simulink model "QuarterCar"  (R2021b)
settings: Solver=ode1  StartTime=0.0  StopTime=inf  FixedStep=0.001  RelTol=1e-3
model workspace (MAT data in the model file):
  Sig = Simulink.Signal
  Sig.DataType = 'auto'
  Sig.Dimensions = -1
  Sig.DimensionsMode = 'auto'
  Sig.Complexity = 'auto'
  Sig.SampleTime = -1
  Sig.SamplingMode = 'auto'
  Sig1 = Simulink.Signal
  Sig1.DataType = 'auto'
  Sig1.Dimensions = -1
  Sig1.DimensionsMode = 'auto'
  Sig1.Complexity = 'auto'
  Sig1.SampleTime = -1
  Sig1.SamplingMode = 'auto'
  Sig2 = Simulink.Signal
  Sig2.DataType = 'auto'
  Sig2.Dimensions = -1
  Sig2.DimensionsMode = 'auto'
  Sig2.Complexity = 'auto'
  Sig2.SampleTime = -1
  Sig2.SamplingMode = 'auto'
undefined symbols (not defined in the file): c_susp, c_tire, g, k_susp, k_tire, m_sprung, m_unsprung, X_sprung0, X_unsprung0
settings Model: Creator=jalfonso  LastModifiedBy=au602135
settings SolverCC: AlgebraicLoopSolver=TrustRegion
settings DataIOCC: ReturnWorkspaceOutputs=off
settings DebuggingCC: SFMachineParentedDataDiag=warning  ArithmeticOperatorsInVariantConditions=warning
settings SFSimCC: SimUseLocalCustomCode=off  CustomCodeUndefinedFunction=UseInterfaceOnly
settings RTWCC: RTWUseLocalCustomCode=off
settings CodeAppCC: StateflowObjectComments=on

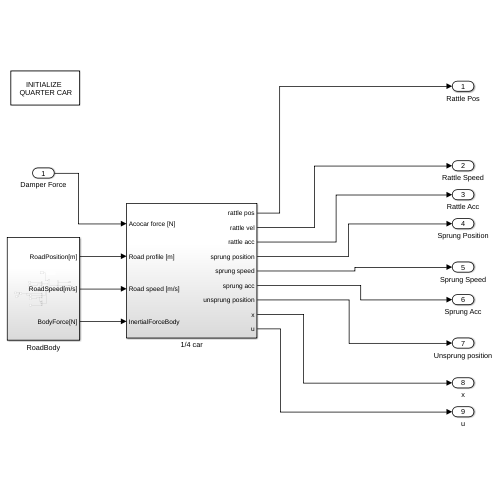
[thumbnail: Simulink's stored preview of the top-level diagram]
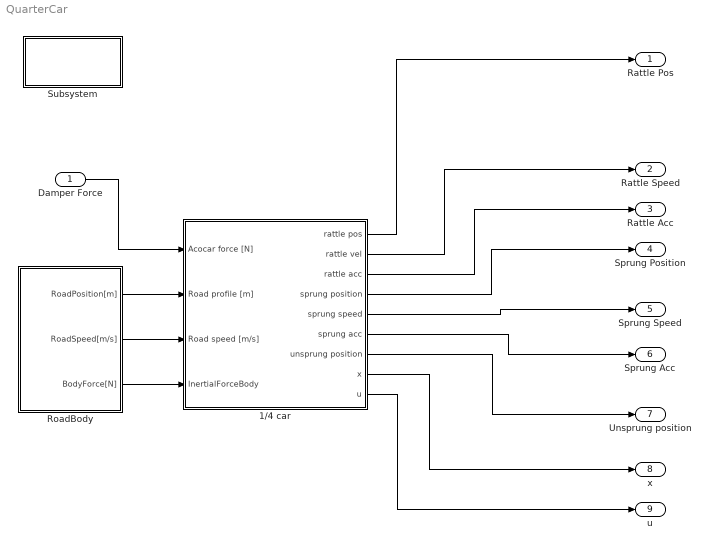
== system QuarterCar ==
  Damper Force : Inport
  1/4 car : Subsystem
  RoadBody : Subsystem
  Subsystem : Subsystem
      settings: OpenFcn=|
      | k_tire = 225400;  %200000 in literature
      | c_tire = 100;        % Estimated. In literatures 6N
      | k_susp =  25000;  % 15000 in literature
      | c_susp = 400;       %1429 Ns/m in literature
      | g = 0 % 9.8; Removed to avoid initialization problems
      | m_unsprung = 66;
      | m_sprung = 449.25;
      | X_sprung0  = .5;
      | X_unsprung0  = .1;
      | delayTimeCarToDamper =  0.002;
      | %InitQuarterCarCompensatorScript;
      | %Amplitude =.01;
      mask Display: disp('INITIALIZE \n QUARTER CAR')
  Rattle Pos : Outport
  Rattle Speed : Outport  Port=2
  Rattle Acc : Outport  Port=3
  Sprung Position : Outport  Port=4
  Sprung Speed : Outport  Port=5
  Sprung Acc : Outport  Port=6
  Unsprung position : Outport  Port=7
  x : Outport  Port=8
  u : Outport  Port=9
  wires:
  RoadBody/1(RoadPosition[m]) -> 1/4 car/2(Road profile [m])
  RoadBody/3(BodyForce[N]) -> 1/4 car/4(InertialForceBody)
  RoadBody/2(RoadSpeed[m/s]) -> 1/4 car/3(Road speed [m/s])
  Damper Force/1 -> 1/4 car/1(Acocar force [N])
  1/4 car/1(rattle pos) -> Rattle Pos/1
  1/4 car/2(rattle vel) -> Rattle Speed/1
  1/4 car/3(rattle acc) -> Rattle Acc/1
  1/4 car/4(sprung position) -> Sprung Position/1
  1/4 car/5(sprung speed) -> Sprung Speed/1
  1/4 car/6(sprung acc) -> Sprung Acc/1
  1/4 car/7(unsprung position) -> Unsprung position/1
  1/4 car/8(x) -> x/1
  1/4 car/9(u) -> u/1

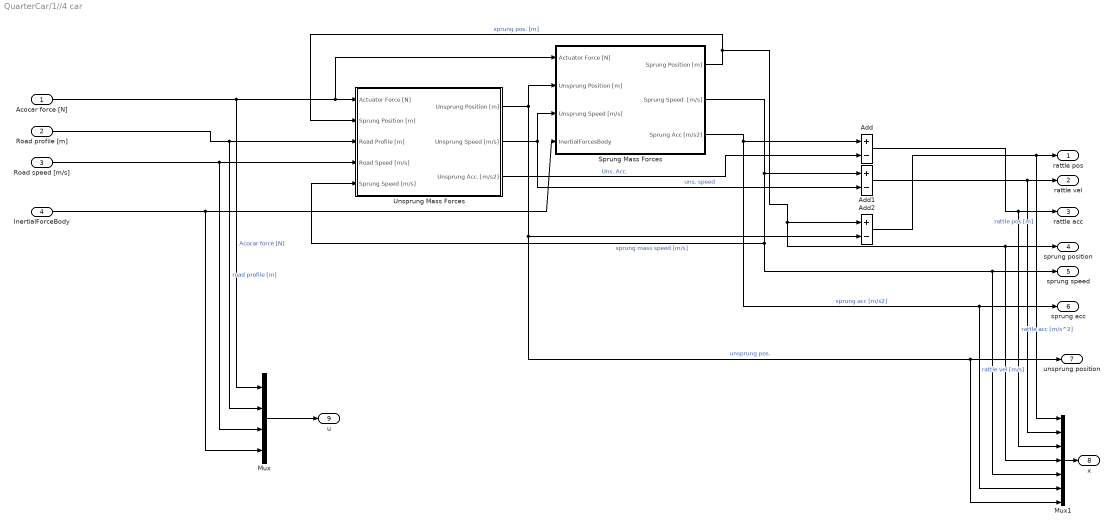
== system QuarterCar/1//4 car ==
  Acocar force [N] : Inport
  Road profile [m] : Inport  Port=2
  Road speed [m/s] : Inport  Port=3
  InertialForceBody : Inport  Port=4
  Add : Sum  Inputs=+-
  Add1 : Sum  Inputs=+-
  Add2 : Sum  Inputs=+-
  Mux : Mux
  Mux1 : Mux  Inputs=7
  Sprung Mass Forces : Subsystem
  Unsprung Mass Forces : Subsystem
  rattle pos : Outport
  rattle vel : Outport  Port=2
  rattle acc : Outport  Port=3
  sprung position : Outport  Port=4
  sprung speed : Outport  Port=5
  sprung acc : Outport  Port=6
  unsprung position : Outport  Port=7
  x : Outport  Port=8
  u : Outport  Port=9
  wires:
  Acocar force [N]/1 -> Mux/1, Sprung Mass Forces/1(Actuator Force [N]), Unsprung Mass Forces/1(Actuator Force [N])  "Acocar force [N]"
  Unsprung Mass Forces/1(Unsprung Position [m]) -> Sprung Mass Forces/2(Unsprung Position [m]), Mux1/7, unsprung position/1, Add2/2  "unsprung pos."
  Unsprung Mass Forces/2(Unsprung Speed [m/s]) -> Sprung Mass Forces/3(Unsprung Speed [m/s]), Add1/2  "uns. speed"
  Sprung Mass Forces/2(Sprung Speed  [m/s]) -> Mux1/5, sprung speed/1, Unsprung Mass Forces/5(Sprung Speed [m/s]), Add1/1  "sprung mass speed [m/s]"
  Sprung Mass Forces/1(Sprung Position [m]) -> Add2/1, Mux1/4, sprung position/1, Unsprung Mass Forces/2(Sprung Position [m])  "sprung pos. [m]"
  Road profile [m]/1 -> Mux/2, Unsprung Mass Forces/3(Road Profile [m])  "road profile [m]"
  Sprung Mass Forces/3(Sprung Acc [m/s2]) -> Mux1/6, sprung acc/1, Add/1  "sprung acc [m/s2]"
  Unsprung Mass Forces/3(Unsprung Acc. [m/s2]) -> Add/2  "Uns. Acc."
  Add/1 -> Mux1/3, rattle acc/1  "rattle acc [m/s^2]"
  Add2/1 -> Mux1/1, rattle pos/1  "rattle pos [m]"
  Add1/1 -> Mux1/2, rattle vel/1  "rattle vel [m/s]"
  Road speed [m/s]/1 -> Mux/3, Unsprung Mass Forces/4(Road Speed [m/s])
  InertialForceBody/1 -> Mux/4, Sprung Mass Forces/4(InertialForcesBody)
  Mux/1 -> u/1
  Mux1/1 -> x/1

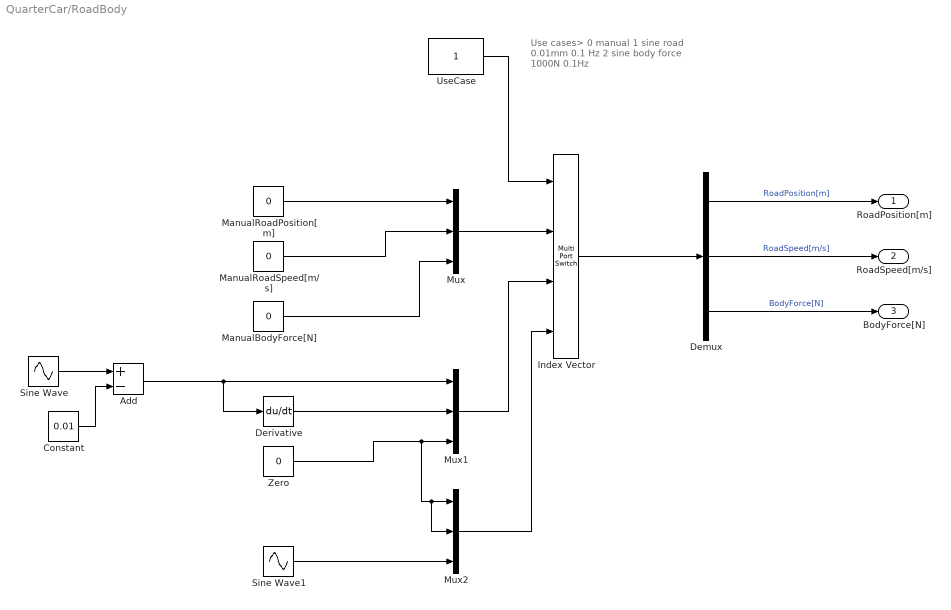
== system QuarterCar/RoadBody ==
  note: Use cases>
      |  0  manual
      | 1 sine road 0.01mm 0.1 Hz
      | 2 sine body force 1000N 0.1Hz
  Add : Sum  Inputs=+-
  Constant : Constant  Value=0.01
  Demux : Demux  Outputs=3
  Derivative : Derivative
  Index Vector : MultiPortSwitch  DataPortOrder=Zero-based contiguous  zeroidx=on
  ManualBodyForce[N] : Constant  Value=0
  ManualRoadPosition[m] : Constant  Value=0
  ManualRoadSpeed[m/s] : Constant  Value=0
  Mux : Mux  Inputs=3
  Mux1 : Mux  Inputs=3
  Mux2 : Mux  Inputs=3
  Sine Wave : Sin  Amplitude=0.01  Frequency=5*(2*pi)  Phase=pi/2  SampleTime=0
  Sine Wave1 : Sin  Amplitude=0.01  Frequency=0.2*pi  SampleTime=0
  UseCase : Constant
  Zero : Constant  Value=0
  RoadPosition[m] : Outport
  RoadSpeed[m/s] : Outport  Port=2
  BodyForce[N] : Outport  Port=3
  wires:
  Derivative/1 -> Mux1/2
  ManualRoadSpeed[m/s]/1 -> Mux/2
  ManualBodyForce[N]/1 -> Mux/3
  ManualRoadPosition[m]/1 -> Mux/1
  Add/1 -> Mux1/1, Derivative/1
  UseCase/1 -> Index Vector/1
  Mux/1 -> Index Vector/2
  Zero/1 -> Mux2/2, Mux2/1, Mux1/3
  Mux1/1 -> Index Vector/3
  Sine Wave1/1 -> Mux2/3
  Mux2/1 -> Index Vector/4
  Demux/2 -> RoadSpeed[m/s]/1  "RoadSpeed[m/s]"
  Demux/1 -> RoadPosition[m]/1  "RoadPosition[m]"
  Demux/3 -> BodyForce[N]/1  "BodyForce[N]"
  Index Vector/1 -> Demux/1
  Sine Wave/1 -> Add/1
  Constant/1 -> Add/2

== system QuarterCar/Subsystem ==

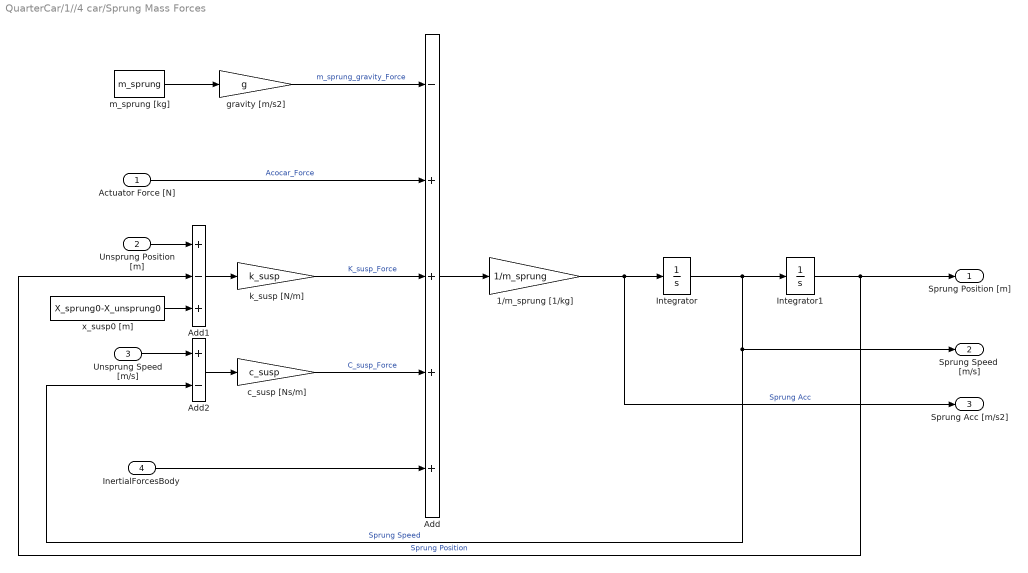
== system QuarterCar/1//4 car/Sprung Mass Forces ==
  Actuator Force [N] : Inport
  Unsprung Position [m] : Inport  Port=2
  Unsprung Speed [m/s] : Inport  Port=3
  InertialForcesBody : Inport  Port=4
  1/m_sprung [1/kg] : Gain  Gain=1/m_sprung
  Add : Sum  Inputs=-++++
  Add1 : Sum  Inputs=+-+
  Add2 : Sum  Inputs=+-
  Integrator : Integrator
  Integrator1 : Integrator  InitialCondition=X_sprung0  UpperSaturationLimit=0.5  LowerSaturationLimit=-0.1
  c_susp [Ns/m] : Gain  Gain=c_susp
  gravity [m/s2] : Gain  Gain=g
  k_susp [N/m] : Gain  Gain=k_susp
  m_sprung [kg] : Constant  Value=m_sprung
  x_susp0 [m] : Constant  Value=X_sprung0-X_unsprung0
  Sprung Position [m] : Outport
  Sprung Speed  [m/s] : Outport  Port=2
  Sprung Acc [m/s2] : Outport  Port=3
  wires:
  1/m_sprung [1/kg]/1 -> Integrator/1, Sprung Acc [m/s2]/1  "Sprung Acc"
  Add/1 -> 1/m_sprung [1/kg]/1
  Add1/1 -> k_susp [N/m]/1
  Add2/1 -> c_susp [Ns/m]/1
  c_susp [Ns/m]/1 -> Add/4  "C_susp_Force"
  Actuator Force [N]/1 -> Add/2  "Acocar_Force"
  k_susp [N/m]/1 -> Add/3  "K_susp_Force"
  Integrator1/1 -> Add1/2, Sprung Position [m]/1  "Sprung Position"
  Integrator/1 -> Integrator1/1, Add2/2, Sprung Speed  [m/s]/1  "Sprung Speed"
  Unsprung Speed [m/s]/1 -> Add2/1
  Unsprung Position [m]/1 -> Add1/1
  gravity [m/s2]/1 -> Add/1  "m_sprung_gravity_Force"
  m_sprung [kg]/1 -> gravity [m/s2]/1
  x_susp0 [m]/1 -> Add1/3
  InertialForcesBody/1 -> Add/5

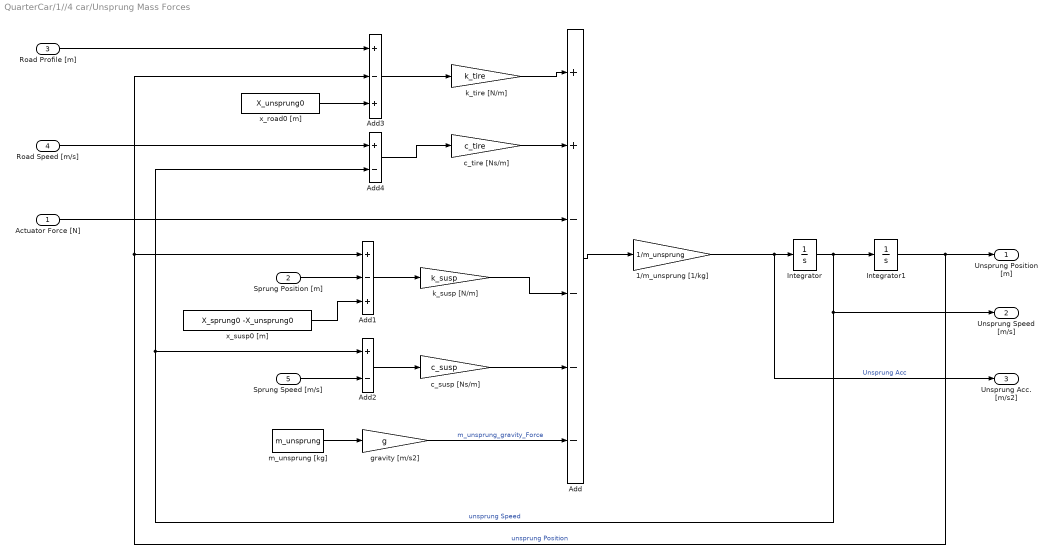
== system QuarterCar/1//4 car/Unsprung Mass Forces ==
  Actuator Force [N] : Inport
  Sprung Position [m] : Inport  Port=2
  Road Profile [m] : Inport  Port=3
  Road Speed [m/s] : Inport  Port=4
  Sprung Speed [m/s] : Inport  Port=5
  1/m_unsprung [1/kg] : Gain  Gain=1/m_unsprung
  Add : Sum  Inputs=++----
  Add1 : Sum  Inputs=+-+
  Add2 : Sum  Inputs=+-
  Add3 : Sum  Inputs=+-+
  Add4 : Sum  Inputs=+-
  Integrator : Integrator
  Integrator1 : Integrator  InitialCondition=X_unsprung0  UpperSaturationLimit=0.2  LowerSaturationLimit=0
  c_susp [Ns/m] : Gain  Gain=c_susp
  c_tire [Ns/m] : Gain  Gain=c_tire
  gravity [m/s2] : Gain  Gain=g
  k_susp [N/m] : Gain  Gain=k_susp
  k_tire [N/m] : Gain  Gain=k_tire
  m_unsprung [kg] : Constant  Value=m_unsprung
  x_road0 [m] : Constant  Value=X_unsprung0
  x_susp0 [m] : Constant  Value=X_sprung0 -X_unsprung0
  Unsprung Position [m] : Outport
  Unsprung Speed [m/s] : Outport  Port=2
  Unsprung Acc. [m/s2] : Outport  Port=3
  wires:
  1/m_unsprung [1/kg]/1 -> Integrator/1, Unsprung Acc. [m/s2]/1  "Unsprung Acc"
  Add/1 -> 1/m_unsprung [1/kg]/1
  Actuator Force [N]/1 -> Add/3
  k_tire [N/m]/1 -> Add/1
  Sprung Position [m]/1 -> Add1/2
  Add1/1 -> k_susp [N/m]/1
  k_susp [N/m]/1 -> Add/4
  Sprung Speed [m/s]/1 -> Add2/2
  Add2/1 -> c_susp [Ns/m]/1
  c_susp [Ns/m]/1 -> Add/5
  Add3/1 -> k_tire [N/m]/1
  Road Profile [m]/1 -> Add3/1
  m_unsprung [kg]/1 -> gravity [m/s2]/1
  gravity [m/s2]/1 -> Add/6  "m_unsprung_gravity_Force"
  x_susp0 [m]/1 -> Add1/3
  x_road0 [m]/1 -> Add3/3
  Integrator1/1 -> Add1/1, Add3/2, Unsprung Position [m]/1  "unsprung Position"
  Integrator/1 -> Integrator1/1, Add2/1, Add4/2, Unsprung Speed [m/s]/1  "unsprung Speed"
  c_tire [Ns/m]/1 -> Add/2
  Add4/1 -> c_tire [Ns/m]/1
  Road Speed [m/s]/1 -> Add4/1
